simulink model "testsloptim"  (Simulink 5.0)
settings: Solver=ode45  StartTime=0  StopTime=100  RelTol=1e-3
values from neighbouring files (symbols this model uses):
  b = {b(1) , b(2)}    [randunc.m]
undefined symbols (not defined in the file or in its folder): a, c
settings Model: Creator=ksubbara  LastModifiedBy=ksubbara

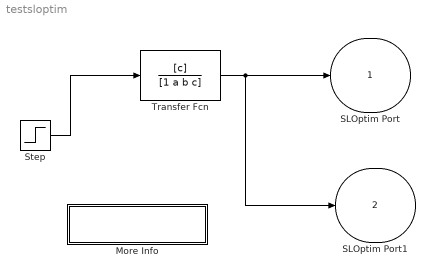
== system testsloptim ==
  More Info : Subsystem
      settings: OpenFcn=a = 0.01; b = 1; c = 0.1;
      mask Display: disp('Intialize Parameters')
  Step : Step  Time=0  SampleTime=0
  Transfer Fcn : TransferFcn  Numerator=[c]  Denominator=[1 a b c]
  SLOptim Port : Outport  InitialOutput=0  mask(SLOptim Port){GUIlocation=[0.15 0.25 0.7 0.5]}
      settings: ModelCloseFcn=sloptimModelClose  PreSaveFcn=sloptimguilocation  OpenFcn=slparoptim;
      mask Display:
      | plot([0:10],[-.5 1.5 .6 1.3 .8 1.1 .95 1.02 .99 1 1])
      | disp(['\n SLOptim_Port',get_param(gcb,'Port')]);
  SLOptim Port1 : Outport  Port=2  InitialOutput=0  mask(SLOptim Port){GUIlocation=[0.15 0.25 0.7 0.5]}
      settings: ModelCloseFcn=sloptimModelClose  PreSaveFcn=sloptimguilocation  OpenFcn=slparoptim;
      mask Display:
      | plot([0:10],[-.5 1.5 .6 1.3 .8 1.1 .95 1.02 .99 1 1])
      | disp(['\n SLOptim_Port',get_param(gcb,'Port')]);
  wires:
  Transfer Fcn/1 -> SLOptim Port1/1, SLOptim Port/1
  Step/1 -> Transfer Fcn/1

== system testsloptim/More Info ==
  note: Merge Block Demonstration
  note: This demonstration shows what happens when the output of two enabled
      | subsystems are merged together.  The output of the merge block is the last
      |  output written to the input ports of the block.
      |
      | While the simulation is running, the subsystem which is green is the one
      | whose signal is displayed on the scope. The coloring of the blocks is
      | controlled by an S-Function which exists in the enabled subsystems.  This
      | S-Function also artifically slows down the simulation by placing a short
      | pause in the S-Function.
